simulink model "motorfault"  (R2022a)
settings: Solver=VariableStepAuto  StartTime=0.0  StopTime=1  RelTol=1e-3
undefined symbols (not defined in the file or in its folder): T
libraries: spsAsynchronousMachineSIUnitsLib x1, spsThreePhaseBreakerLib x1, spsThreePhaseFaultLib x1, spsThreePhaseSourceLib x1, spsVoltageMeasurementLib x1, spspowerguiLib x1
settings Model: Creator=Edwin  LastModifiedBy=Edwin

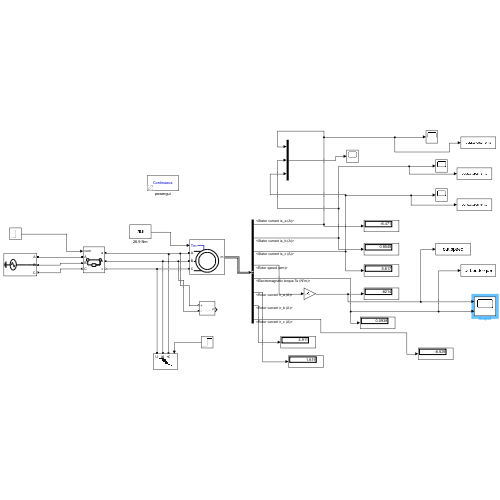
[thumbnail: Simulink's stored preview of the top-level diagram]
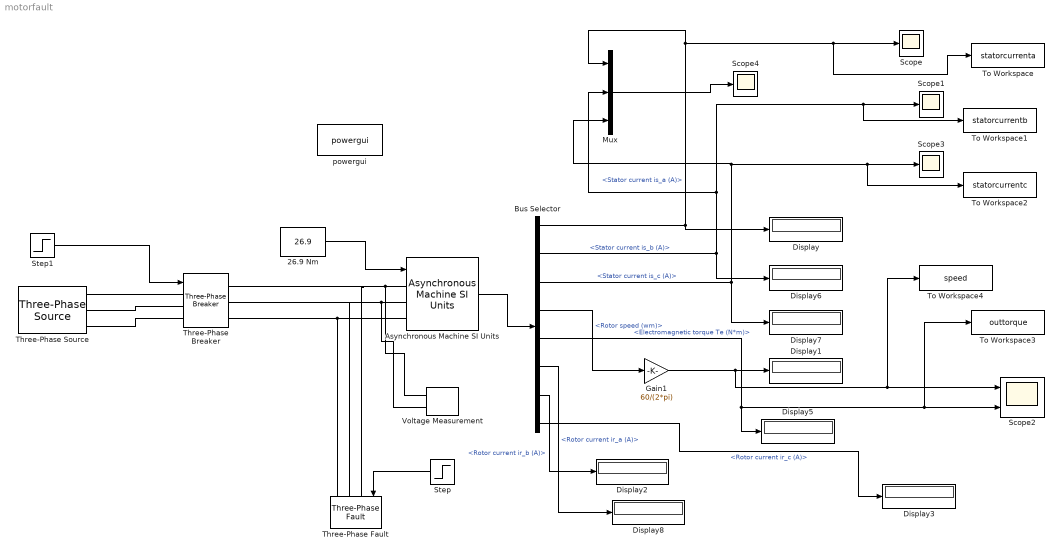
== system motorfault ==
  26.9 Nm : Constant  Value=26.9
  Asynchronous Machine SI Units : spsAsynchronousMachineSIUnitsLib/Asynchronous Machine SI Units  RotorType=Squirrel-cage  PresetModel="15:  5.4 HP (4KW)   400 V  50Hz 1430 RPM"  MechanicalLoad=Torque Tm  ShowDetailedParameters=on  ReferenceFrame=Rotor  Units=SI  MeasurementBus=off  NominalParameters=[4000 400 50]  VoltageRatio=1  Stator=[1.405 0.005839]  Rotor=[1.395 0.005839]  Cage1=[0.4155 0.002066]  Cage2=[0.4168 0.0003495]  Lm=0.1722  Mechanical=[0.0131 0.002985 2]  PolePairs=2  InitialConditions=[0 0 0 0 0 0 0 0]  SimulateSaturation=off  Saturation=[14.03593122, 27.81365428, 53.79336849, 72.68890987, 97.98006896, 148.6815601, 215.7428561, 302.9841135, 428.7778367 ; 230, 322, 414, 460, 506, 552, 598, 644, 690]  LoadFlowParameters=1492000  TsPowergui=0  TsBlock=-1  IterativeModel=Trapezoidal non iterative  IterativeDiscreteModel=Trapezoidal non iterative  Pmec=1.492e+006
  Bus Selector : BusSelector  OutputSignals=Stator measurements.Stator current is_a (A),Stator measurements.Stator current is_b (A),Stator measurements.Stator current is_c (A),Mechanical.Rotor speed (wm),Mechanical.Electromagnetic torque Te (N*m),Rotor measurements.Rotor current ir_a (A),Rotor measurements.Rotor current ir_b (A),Rotor measurements.Rotor current ir_c (A)
  Display{,1..3,5..8} (8 alike) : Display
  Gain1 : Gain  Gain=60/(2*pi)
  Mux : Mux  Inputs=3
  Scope{,1,3..4} (4 alike) : Scope
  Scope2 : Scope  NumInputPorts=2
  Step : Step  Time=0.5  SampleTime=0
  Step1 : Step  Time=5  Before=1  SampleTime=0
  Three-Phase Breaker : spsThreePhaseBreakerLib/Three-Phase Breaker  InitialState=closed  SwitchA=on  SwitchB=on  SwitchC=on  SwitchTimes="[1/60  5/60]"  External=on  BreakerResistance=0.01  SnubberResistance=1e6  SnubberCapacitance=inf  Measurements=None
  Three-Phase Fault : spsThreePhaseFaultLib/Three-Phase Fault  InitialStates=0  FaultA=on  FaultB=on  FaultC=on  GroundFault=on  SwitchTimes="[1/60  5/60]"  External=on  SwitchStatus=NaN  FaultResistance=0.001  GroundResistance=0.01  SnubberResistance=1e6  SnubberCapacitance=inf  Measurements=None
  Three-Phase Source : spsThreePhaseSourceLib/Three-Phase Source  InternalConnection=Yg  VoltagePhases=off  Voltage=400  PhaseAngle=0  Voltage_phases=[25e3 25e3 25e3]/sqrt(3)  PhaseAngles_phases=[0 -120 +120]  Frequency=50  NonIdealSource=off  SpecifyImpedance=off  Resistance=0.8929  Inductance=16.58e-3  ShortCircuitLevel=100e6  BaseVoltage=25e3  XRratio=7  BusType=swing  Pref=10e3  Qref=0  Prefabc=[10e3, 10e3, 10e3]  Qrefabc=[0, 0, 0]  Qmin=-inf  Qmax=inf
  To Workspace : ToWorkspace  VariableName=statorcurrenta  SampleTime=-1
  To Workspace1 : ToWorkspace  VariableName=statorcurrentb  SampleTime=-1
  To Workspace2 : ToWorkspace  VariableName=statorcurrentc  SampleTime=-1
  To Workspace3 : ToWorkspace  VariableName=outtorque  SampleTime=-1
  To Workspace4 : ToWorkspace  VariableName=speed  SampleTime=-1
  Voltage Measurement : spsVoltageMeasurementLib/Voltage Measurement  PhasorSimulation=off  OutputType=Complex  PSBequivalent=0
  powergui : spspowerguiLib/powergui  Priority=1  SimulationMode=Continuous  SampleTime=T  frequency=60  Iterations=50  frequencyindice=50  Pbase=100e6  ErrMax=1e-4  UnitsV=kV  UnitsW=MW  buscounter=0  FunctionMessages=off  echomessages=off  EnableUseOfTLC=off  CurrentSourceSwitches=off  DisableSnubberDevices=off  DisableRonSwitches=off  DisableVfSwitches=off  DisplayEquations=off  AutomaticDiscreteSolvers=off  SolverType=Tustin/Backward Euler (TBE)  Interpol=off  ExternalGateDelay=off  methode=off  Ts=100  x0status=blocks  SPID=on  SwTol=0  HookPort=off  NonlinearTolerance=1e-4  nMaxIteration=100  ContinueOnMaxIteration=off  RestoreLinks=warning  ResistiveCurrentMeasurement=off  Frange=[0:2:500]  Ylog=off  Xlog=on  ShowGrid=off  save=off  variable=ZData  structure=0  ZoomFFT=off  StartTime=0.0  cycles=1  DisplayStyle=1  fundamental=60  FreqAxis=off  MaxFrequency=1000  frequencyindicesteady=1  RmsSteady=1  display=off
  wires:
  Bus Selector/2 -> Mux/2, To Workspace1/1, Scope1/1, Display6/1  "<Stator current is_b (A)>"
  Gain1/1 -> To Workspace4/1, Scope2/1, Display1/1
  Bus Selector/4 -> Gain1/1  "<Rotor speed (wm)>"
  Asynchronous Machine SI Units/1 -> Bus Selector/1
  Bus Selector/3 -> Mux/3, To Workspace2/1, Scope3/1, Display7/1  "<Stator current is_c (A)>"
  Bus Selector/1 -> Mux/1, To Workspace/1, Scope/1, Display/1  "<Stator current is_a (A)>"
  Step1/1 -> Three-Phase Breaker/1
  Step/1 -> Three-Phase Fault/1
  Bus Selector/5 -> Display5/1, To Workspace3/1, Scope2/2  "<Electromagnetic torque Te (N*m)>"
  26.9 Nm/1 -> Asynchronous Machine SI Units/1
  Bus Selector/6 -> Display8/1  "<Rotor current ir_a (A)>"
  Bus Selector/7 -> Display2/1  "<Rotor current ir_b (A)>"
  Bus Selector/8 -> Display3/1  "<Rotor current ir_c (A)>"
  Mux/1 -> Scope4/1
  connections:
  Voltage Measurement/LConn1 -- Three-Phase Breaker/RConn1 -- Three-Phase Fault/LConn1 -- Asynchronous Machine SI Units/LConn1
  Three-Phase Breaker/RConn3 -- Asynchronous Machine SI Units/LConn3 -- Three-Phase Fault/LConn3
  Voltage Measurement/LConn2 -- Three-Phase Fault/LConn2 -- Three-Phase Breaker/RConn2 -- Asynchronous Machine SI Units/LConn2
  Three-Phase Source/RConn3 -- Three-Phase Breaker/LConn3
  Three-Phase Source/RConn1 -- Three-Phase Breaker/LConn1
  Three-Phase Source/RConn2 -- Three-Phase Breaker/LConn2
